simulink library "LIB_CycleControl"  (R2018b)
settings: Solver=VariableStepAuto  StartTime=0.0  StopTime=10.0  RelTol=1e-3
undefined symbols (not defined in the file or in its folder): eActuators, eRespiratorStates, NActuatorActive, nBlowerCmdInit, nBlowerCmdMax, nBlowerCmdMin, nBlowerDecHigh, nBlowerDecMedium, nBlowerIncHigh, nBlowerIncLow, nBlowerIncMedium, NBlowerSpeedIncCorrectionGain, NBlowerValveDerivativeGain, NBlowerValveIntegralGain, NBlowerValveIntegralHighGain, NBlowerValvePropGain, NCyclePerMinMax, NCyclePerMinMin, NMaxPressureSample, NPatientValveDerivativeGain, NPatientValveIntegralGain, NPatientValveIntegralHighGain, NPatientValvePropGain, pBlowerValveOutletOffset, pDiffMaxThdForPlateauPlausibility, pDiffThdForBlowerValveControlActivation, pDiffThdForPatientValveControlActivation, pErrorPlausibilityThd, pErrorThdForHighBlowerDec, pStaticErrorThdForHighBlowerInc, rPIDIntegralMaxTermForBlowerValve, rPIDIntegralMaxTermForPatientValve, rPIDIntegralMinTermForBlowerValve, rPIDIntegralMinTermForPatientValve, tBlowerValveOpen, tDelayBeforeRespiratorCycleStart, tDelayForRespiratorStop, tPatientValveOpen, tPhase1Ofs, tStopInhalationPhase1Min
libraries: simulink x62, simulink_need_slupdate x4, simulink_extras x3
(part 2 of 4)

== system LIB_CycleControl/Cycle Control/Cycle Control Wrapper/Cycle pController/Pressure processing/PPep Computation ==
  BInitCyclePressure [-] : Inport
  NRespiratorCycleStatus [-] : Inport  Port=2
  pBlowerValveOutletLastValuesMean [mmH2O] : Inport  Port=3
  Compare To Constant4 : simulink/Logic and Bit Operations/Compare To Constant  relop===  const=eRespiratorStates.NRespiratorInExhalation  OutDataTypeStr=boolean
  Data Store Write1 : DataStoreWrite  DataStoreName=pBlowerValveOutletExhalationCurrent
  Logical Operator7 : Logic  Operator=OR  AllPortsSameDT=off  OutDataTypeStr=boolean
  PPep Computation : Subsystem
  pBlowerValveOutletExhalationCurrent [mmH2O] : Outport
  wires:
  pBlowerValveOutletLastValuesMean [mmH2O]/1 -> PPep Computation/2(pBlowerValveOutletLastValuesMean [mmH2O])
  BInitCyclePressure [-]/1 -> Logical Operator7/2, PPep Computation/1(BInitCyclePressure [-])
  Compare To Constant4/1 -> Logical Operator7/1
  Logical Operator7/1 -> PPep Computation/Enable
  PPep Computation/1(pBlowerValveOutletExhalationCurrent [mmH2O]) -> pBlowerValveOutletExhalationCurrent [mmH2O]/1, Data Store Write1/1  "pBlowerValveOutletExhalationCurrent"
  NRespiratorCycleStatus [-]/1 -> Compare To Constant4/1

== system LIB_CycleControl/Cycle Control/Cycle Control Wrapper/Cycle pController/Pressure processing/PPlateau Computation ==
  BInitCyclePressure [-] : Inport
  NRespiratorCycleStatus [-] : Inport  Port=2
  pBlowerValveOutletLastValuesMax [mmH2O] : Inport  Port=3
  pBlowerValveOutletLastValuesMin [mmH2O] : Inport  Port=4
  pBlowerValveOutletLastValuesMean [mmH2O] : Inport  Port=5
  Compare To Constant6 : simulink/Logic and Bit Operations/Compare To Constant  relop===  const=eRespiratorStates.NRespiratorInInhalationPhase2  OutDataTypeStr=boolean
  Data Store Write1 : DataStoreWrite  DataStoreName=BpBlowerValveOutletPlateauStabilized
  Data Store Write3 : DataStoreWrite  DataStoreName=pBlowerValveOutletPlateauCurrent
  Logical Operator7 : Logic  Operator=OR  AllPortsSameDT=off  OutDataTypeStr=boolean
  Plateau Compute : Subsystem
  pBlowerValveOutletPlateauCurrent [mmH2O] : Outport
  BpBlowerValveOutletPlateauStabilized [-] : Outport  Port=2
  wires:
  Plateau Compute/2(BpBlowerValveOutletPlateauStabilized [-]) -> BpBlowerValveOutletPlateauStabilized [-]/1, Data Store Write1/1  "BpBlowerValveOutletPlateauStabilized"
  pBlowerValveOutletLastValuesMean [mmH2O]/1 -> Plateau Compute/4(pBlowerValveOutletLastValuesMean [mmH2O])
  pBlowerValveOutletLastValuesMin [mmH2O]/1 -> Plateau Compute/3(pBlowerValveOutletLastValuesMin [mmH2O])
  pBlowerValveOutletLastValuesMax [mmH2O]/1 -> Plateau Compute/2(pBlowerValveOutletLastValuesMax [mmH2O])
  Logical Operator7/1 -> Plateau Compute/Enable
  Compare To Constant6/1 -> Logical Operator7/2
  [BInitCyclePressure] -> Plateau Compute/1(BInitCyclePressure [-])
  NRespiratorCycleStatus [-]/1 -> Compare To Constant6/1
  [BInitCyclePressure] -> Logical Operator7/1
  BInitCyclePressure [-]/1 -> [BInitCyclePressure]
  Plateau Compute/1(pBlowerValveOutletPlateauCurrent [mmH2O]) -> pBlowerValveOutletPlateauCurrent [mmH2O]/1, Data Store Write3/1  "pBlowerValveOutletPlateauCurrent"

== system LIB_CycleControl/Cycle Control/Cycle Control Wrapper/Cycle pController/Pressure processing/PPlateau Error Max Computation ==
  BInitCyclePressure [-] : Inport
  NRespiratorCycleStatus [-] : Inport  Port=2
  pBlowerValveOutletPeakCurrent [mmH2O] : Inport  Port=3
  pBlowerValveOutlet [mmH2O] : Inport  Port=4
  pBlowerValveOutletPlateauTargetApplied [mmH2O] : Inport  Port=5
  Compare To Constant6 : simulink/Logic and Bit Operations/Compare To Constant  relop===  const=eRespiratorStates.NRespiratorInInhalationPhase2  OutDataTypeStr=boolean
  Data Store Write3 : DataStoreWrite  DataStoreName=pBlowerValveOutletErrorMaxCurrent
  Error Compute : Subsystem
  Logical Operator1 : Logic  AllPortsSameDT=off  OutDataTypeStr=boolean
  Logical Operator7 : Logic  Operator=OR  AllPortsSameDT=off  OutDataTypeStr=boolean
  Relational Operator : RelationalOperator  Operator=>  OutDataTypeStr=boolean  RndMeth=Simplest
  Unit Delay : UnitDelay  SampleTime=-1
      settings: AttributesFormatString=%<InitialCondition>
  pBlowerValveOutletErrorMaxCurrent [mmH2O] : Outport
  wires:
  [pBlowerValveOutlet] -> Error Compute/3(pBlowerValveOutlet [mmH2O])
  Unit Delay/1 -> Error Compute/4(pBlowerValveOutletErrorMaxCurrentPrev [mmH2O])
  [pBlowerValveOutletPlateauTargetApplied] -> Error Compute/2(pBlowerValveOutletPlateauTargetApplied [mmH2O])
  Relational Operator/1 -> Logical Operator1/2
  [pBlowerValveOutletPeakCurrent] -> Relational Operator/1
  [pBlowerValveOutletPlateauTargetApplied] -> Relational Operator/2
  pBlowerValveOutletPeakCurrent [mmH2O]/1 -> [pBlowerValveOutletPeakCurrent]
  pBlowerValveOutletPlateauTargetApplied [mmH2O]/1 -> [pBlowerValveOutletPlateauTargetApplied]
  Logical Operator1/1 -> Logical Operator7/2
  Compare To Constant6/1 -> Logical Operator1/1
  pBlowerValveOutlet [mmH2O]/1 -> [pBlowerValveOutlet]
  Logical Operator7/1 -> Error Compute/Enable
  [BInitCyclePressure] -> Error Compute/1(BInitCyclePressure [-])
  NRespiratorCycleStatus [-]/1 -> Compare To Constant6/1
  [BInitCyclePressure] -> Logical Operator7/1
  BInitCyclePressure [-]/1 -> [BInitCyclePressure]
  Error Compute/1(pBlowerValveOutletErrorMaxCurrent [mmH2O]) -> pBlowerValveOutletErrorMaxCurrent [mmH2O]/1, Data Store Write3/1, Unit Delay/1  "pBlowerValveOutletErrorMaxCurrent"

== system LIB_CycleControl/Cycle Control/Cycle Control Wrapper/Cycle pController/Pressure processing/Pressure Release  ==
  NRespiratorCycleStatus [-] : Inport
  BInitCyclePressure [-] : Inport  Port=2
  pBlowerValveOutletPeakCurrentPrev [mmH2O] : Inport  Port=3
  pBlowerValveOutletErrorMaxCurrentPrev [mmH2O] : Inport  Port=4
  pBlowerValveOutletPlateauCurrentPrev [mmH2O] : Inport  Port=5
  BpBlowerValveOutletPlateauStabilizedPrev [-] : Inport  Port=6
  pBlowerValveOutletExhalationCurrentPrev [mmH2O] : Inport  Port=7
  Release : Subsystem
  pBlowerValveOutletPeakLastCycle [mmH2O] : Outport
  pBlowerValveOutletPlateauLastCycle [mmH2O] : Outport  Port=2  InitialOutput=0
  pBlowerValveOutletEndLastCycle [mmH2O] : Outport  Port=3
  pBlowerValveOutletErrorMaxLastCycle [mmH2O] : Outport  Port=4  InitialOutput=0
  wires:
  Release/3(pBlowerValveOutletEndLastCycle [mmH2O]) -> pBlowerValveOutletEndLastCycle [mmH2O]/1
  Release/1(pBlowerValveOutletPeakLastCycle [mmH2O]) -> pBlowerValveOutletPeakLastCycle [mmH2O]/1
  BpBlowerValveOutletPlateauStabilizedPrev [-]/1 -> Release/6(BpBlowerValveOutletPlateauStabilizedPrev [-])
  pBlowerValveOutletErrorMaxCurrentPrev [mmH2O]/1 -> Release/5(pBlowerValveOutletErrorMaxCurrentPrev [mmH2O])
  Release/4(pBlowerValveOutletErrorMaxLastCycle [mmH2O]) -> pBlowerValveOutletErrorMaxLastCycle [mmH2O]/1
  BInitCyclePressure [-]/1 -> Release/Enable
  Release/2(pBlowerValveOutletPlateauLastCycle [mmH2O]) -> pBlowerValveOutletPlateauLastCycle [mmH2O]/1
  pBlowerValveOutletExhalationCurrentPrev [mmH2O]/1 -> Release/4(pBlowerValveOutletExhalationCurrentPrev [mmH2O])
  pBlowerValveOutletPlateauCurrentPrev [mmH2O]/1 -> Release/3(pBlowerValveOutletPlateauCurrentPrev [mmH2O])
  pBlowerValveOutletPeakCurrentPrev [mmH2O]/1 -> Release/2(pBlowerValveOutletPeakCurrentPrev [mmH2O])
  NRespiratorCycleStatus [-]/1 -> Release/1(NRespiratorCycleStatus [-])

== system LIB_CycleControl/Cycle Control/Cycle Control Wrapper/Cycle pController/Pressure processing/Pressure recording Update ==
  note: [0...NSample-1]
  pBlowerValveOutlet [mmH2O] : Inport
  BInitCyclePressure [-] : Inport  Port=2
  Assignment : Assignment  IndexMode=Zero-based  DiagnosticForDimensions=Warning  IndexOptions=Index vector (port)  Indices=1  OutputSizes=1
      settings: AttributesFormatString=%<IndexMode>
  Constant : Constant  Value=zeros(1,NMaxPressureSample)  OutDataTypeStr=single
  Constant1 : Constant  Value=NMaxPressureSample
  Counter : Subsystem
  Data Store Write1 : DataStoreWrite  DataStoreName=pBlowerValveOutletLastValuesMin
  Data Store Write2 : DataStoreWrite  DataStoreName=pBlowerValveOutletLastValuesMax
  Data Store Write3 : DataStoreWrite  DataStoreName=pBlowerValveOutletLastValuesMean
  MinMax : MinMax  Function=max
  MinMax1 : MinMax
  Product : Product  Inputs=*/
  Sum of Elements : Sum  Inputs=+
  Switch4 : Switch  Criteria=u2 ~= 0
      settings: AttributesFormatString=%<Criteria>
  Unit Delay : UnitDelay  InitialCondition=zeros(1,NMaxPressureSample)  SampleTime=-1
      settings: AttributesFormatString=%<InitialCondition>
  pBlowerValveOutletLastValuesMax [mmH2O] : Outport
  pBlowerValveOutletLastValuesMin [mmH2O] : Outport  Port=2
  pBlowerValveOutletLastValuesMean [mmH2O] : Outport  Port=3
  wires:
  Product/1 -> pBlowerValveOutletLastValuesMean [mmH2O]/1, Data Store Write3/1  "pBlowerValveOutletLastValuesMean"
  MinMax1/1 -> pBlowerValveOutletLastValuesMin [mmH2O]/1, Data Store Write1/1  "pBlowerValveOutletLastValuesMin"
  MinMax/1 -> pBlowerValveOutletLastValuesMax [mmH2O]/1, Data Store Write2/1  "pBlowerValveOutletLastValuesMax"
  Constant1/1 -> Product/2
  Sum of Elements/1 -> Product/1
  pBlowerValveOutlet [mmH2O]/1 -> Assignment/2
  Counter/1(NPressureSampleIndex [-]) -> Assignment/3
  Constant/1 -> Switch4/1
  BInitCyclePressure [-]/1 -> Switch4/2
  Switch4/1 -> MinMax1/1, Sum of Elements/1, Unit Delay/1, MinMax/1
  Assignment/1 -> Switch4/3
  Unit Delay/1 -> Assignment/1

== system LIB_CycleControl/Cycle Control/Cycle Control Wrapper/Cycle pController/ValvePosition_Target/Exhalation ==
  BExternalInit [-] : Inport
  tPeriodTask [s] : Inport  Port=2
  pBlowerValveOutletTarget [mmH2O] : Inport  Port=3
  pBlowerValveOutlet [mmH2O] : Inport  Port=4
  rPatientValveCmdPrev [%] : Inport  Port=5
  Action Port : ActionPort
  Constant2 : Constant  Value=0  OutDataTypeStr=Inherit: Inherit via back propagation
  Patient Valve Control : Subsystem
  Sum : Sum  Inputs=|+-  SaturateOnIntegerOverflow=on
  rBlowerValveCmd [%] : Outport
  rPatientValveCmd [%] : Outport  Port=2
  wires:
  Sum/1 -> Patient Valve Control/4(Error [mmH2O])
  rPatientValveCmdPrev [%]/1 -> Patient Valve Control/5(rPatientValveCmdPrev [%])
  Patient Valve Control/1(rPatientValveCmd [%]) -> rPatientValveCmd [%]/1
  BExternalInit [-]/1 -> Patient Valve Control/2(BExternalInit [-])
  pBlowerValveOutletTarget [mmH2O]/1 -> Sum/1, Patient Valve Control/3(pBlowerValveOutletTarget [mmH2O])
  pBlowerValveOutlet [mmH2O]/1 -> Sum/2
  tPeriodTask [s]/1 -> Patient Valve Control/1(tPeriodTask [s])
  Constant2/1 -> rBlowerValveCmd [%]/1

== system LIB_CycleControl/Cycle Control/Cycle Control Wrapper/Cycle pController/ValvePosition_Target/Inhalation ==
  BExternalInit [-] : Inport
  tPeriodTask [s] : Inport  Port=2
  pBlowerValveOutletTarget [mmH2O] : Inport  Port=3
  pBlowerValveOutlet [mmH2O] : Inport  Port=4
  rBlowerValveCmdPrev [%] : Inport  Port=5
  Action Port : ActionPort
  Blower Valve Control : Subsystem
  Constant9 : Constant  Value=0  OutDataTypeStr=single
  Sum : Sum  Inputs=|+-  SaturateOnIntegerOverflow=on
  rBlowerValveCmd [%] : Outport
  rPatientValveCmd [%] : Outport  Port=2
  wires:
  rBlowerValveCmdPrev [%]/1 -> Blower Valve Control/4(rBlowerValveCmdPrev [%])
  Sum/1 -> Blower Valve Control/3(Error)
  Blower Valve Control/1(rBlowerValveCmd [%]) -> rBlowerValveCmd [%]/1
  pBlowerValveOutlet [mmH2O]/1 -> Sum/2
  tPeriodTask [s]/1 -> Blower Valve Control/1(tPeriodTask [s])
  pBlowerValveOutletTarget [mmH2O]/1 -> Sum/1
  BExternalInit [-]/1 -> Blower Valve Control/2(BExternalInit [-])
  Constant9/1 -> rPatientValveCmd [%]/1

== system LIB_CycleControl/Cycle Control/Cycle Control Wrapper/Cycle pController/ValvePosition_Target/START ==
  Action Port : ActionPort
  Constant2 : Constant  Value=0  OutDataTypeStr=Inherit: Inherit via back propagation
  Constant9 : Constant  Value=100  OutDataTypeStr=Inherit: Inherit via back propagation
  rBlowerValveCmd [%] : Outport
  rPatientValveCmd [%] : Outport  Port=2
  wires:
  Constant2/1 -> rBlowerValveCmd [%]/1
  Constant9/1 -> rPatientValveCmd [%]/1

== system LIB_CycleControl/Cycle Control/Cycle Control Wrapper/Cycle pController/ValvePosition_Target/STOP ==
  tCycle [s] : Inport
  Action Port : ActionPort
  Constant1 : Constant  Value=100  OutDataTypeStr=Inherit: Inherit via back propagation
  Constant2 : Constant  Value=0  OutDataTypeStr=Inherit: Inherit via back propagation
  Constant3 : Constant  Value=tDelayForRespiratorStop  OutDataTypeStr=single
  Constant9 : Constant  Value=100  OutDataTypeStr=single
  Gain : Gain  Gain=0.5
  Relational Operator : RelationalOperator  Operator=>  OutDataTypeStr=boolean  RndMeth=Simplest
  Switch3 : Switch  Criteria=u2 ~= 0
      settings: AttributesFormatString=%<Criteria>
  rBlowerValveCmd [%] : Outport
  rPatientValveCmd [%] : Outport  Port=2
  wires:
  Constant3/1 -> Gain/1
  Constant2/1 -> Switch3/3
  Constant1/1 -> rPatientValveCmd [%]/1
  Gain/1 -> Relational Operator/2
  Switch3/1 -> rBlowerValveCmd [%]/1
  Constant9/1 -> Switch3/1
  Relational Operator/1 -> Switch3/2
  tCycle [s]/1 -> Relational Operator/1

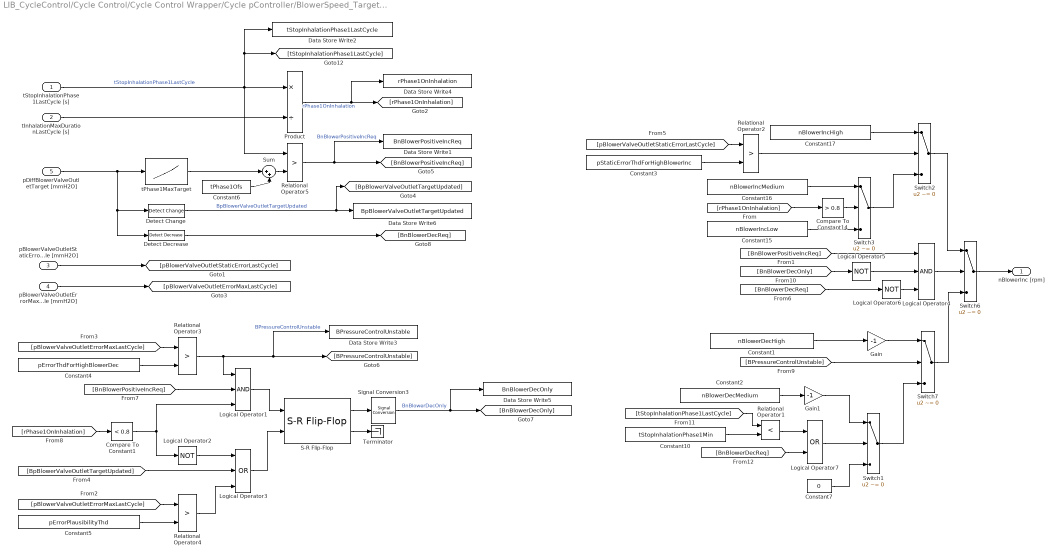
== system LIB_CycleControl/Cycle Control/Cycle Control Wrapper/Cycle pController/BlowerSpeed_Target/CycleStartComputation/Blower Inc from Last Cycle ==
  tStopInhalationPhase1LastCycle [s] : Inport
  tInhalationMaxDurationLastCycle [s] : Inport  Port=2
  "pBlowerValveOutletStaticErrorLastCycle [mmH2O] " : Inport  Port=3
  pBlowerValveOutletErrorMaxLastCycle [mmH2O] : Inport  Port=4
  pDiffBlowerValveOutletTarget [mmH2O] : Inport  Port=5
  Compare To Constant1 : simulink/Logic and Bit Operations/Compare To Constant  relop=<  const=0.8  OutDataTypeStr=boolean
  Compare To Constant14 : simulink/Logic and Bit Operations/Compare To Constant  relop=>  const=0.8  OutDataTypeStr=boolean
  Constant1 : Constant  Value=nBlowerDecHigh  OutDataTypeStr=single
  Constant10 : Constant  Value=tStopInhalationPhase1Min  OutDataTypeStr=single
  Constant15 : Constant  Value=nBlowerIncLow  OutDataTypeStr=single
  Constant16 : Constant  Value=nBlowerIncMedium  OutDataTypeStr=single
  Constant17 : Constant  Value=nBlowerIncHigh  OutDataTypeStr=single
  Constant2 : Constant  Value=nBlowerDecMedium  OutDataTypeStr=single
  Constant3 : Constant  Value=pStaticErrorThdForHighBlowerInc  OutDataTypeStr=single
  Constant4 : Constant  Value=pErrorThdForHighBlowerDec  OutDataTypeStr=single
  Constant5 : Constant  Value=pErrorPlausibilityThd  OutDataTypeStr=single
  Constant6 : Constant  Value=tPhase1Ofs  OutDataTypeStr=single
  Constant7 : Constant  Value=0  OutDataTypeStr=single
  Data Store Write1 : DataStoreWrite  DataStoreName=BnBlowerPositiveIncReq
  Data Store Write2 : DataStoreWrite  DataStoreName=tStopInhalationPhase1LastCycle
  Data Store Write3 : DataStoreWrite  DataStoreName=BPressureControlUnstable
  Data Store Write4 : DataStoreWrite  DataStoreName=rPhase1OnInhalation
  Data Store Write5 : DataStoreWrite  DataStoreName=BnBlowerDecOnly
  Data Store Write6 : DataStoreWrite  DataStoreName=BpBlowerValveOutletTargetUpdated
  Detect Change : simulink/Logic and Bit Operations/Detect Change  vinit=0  OutDataTypeStr=boolean
  Detect Decrease : simulink/Logic and Bit Operations/Detect Decrease  vinit=0.0  OutDataTypeStr=boolean
  Gain : Gain  Gain=-1
  Gain1 : Gain  Gain=-1
  Logical Operator1 : Logic  Inputs=3  AllPortsSameDT=off  OutDataTypeStr=boolean
  Logical Operator2 : Logic  Operator=NOT  Inputs=3  AllPortsSameDT=off  OutDataTypeStr=boolean
  Logical Operator3 : Logic  Operator=OR  Inputs=3  AllPortsSameDT=off  OutDataTypeStr=boolean
  Logical Operator4 : Logic  Inputs=3  AllPortsSameDT=off  OutDataTypeStr=boolean
  Logical Operator5 : Logic  Operator=NOT  Inputs=3  AllPortsSameDT=off  OutDataTypeStr=boolean
  Logical Operator6 : Logic  Operator=NOT  Inputs=3  AllPortsSameDT=off  OutDataTypeStr=boolean
  Logical Operator7 : Logic  Operator=OR  AllPortsSameDT=off  OutDataTypeStr=boolean
  Product : Product  Inputs=*/
  Relational Operator1 : RelationalOperator  Operator=<  OutDataTypeStr=boolean  RndMeth=Simplest
  Relational Operator{2..5} (4 alike) : RelationalOperator  Operator=>  OutDataTypeStr=boolean  RndMeth=Simplest
  S-R Flip-Flop : simulink_extras/Flip Flops/S-R Flip-Flop  initial_condition=0
  Signal Conversion3 : SignalConversion  OverrideOpt=off
  Sum : Sum  Inputs=|++
  Switch{1..3,6..7} (5 alike) : Switch  Criteria=u2 ~= 0
      settings: AttributesFormatString=%<Criteria>
  Terminator : Terminator
  tPhase1MaxTarget : Lookup_n-D  NumberOfTableDimensions=1  BreakpointsForDimension1=[50 100 150 200 250 350]  IndexSearchMethod=Linear search  BeginIndexSearchUsingPreviousIndexResult=on  Table=[0.225 0.275 0.35 0.425 0.55 0.8]  ExtrapMethod=Clip  UseLastTableValue=on  InternalRulePriority=Speed  RndMeth=Simplest  InputSameDT=on
  nBlowerInc [rpm] : Outport
  wires:
  Constant6/1 -> Sum/2
  Sum/1 -> Relational Operator5/2
  tPhase1MaxTarget/1 -> Sum/1
  [BnBlowerDecReq] -> Logical Operator7/2
  Relational Operator1/1 -> Logical Operator7/1
  Logical Operator7/1 -> Switch1/2
  [BPressureControlUnstable] -> Switch7/2
  [BnBlowerDecReq] -> Logical Operator6/1
  Logical Operator6/1 -> Logical Operator4/3
  Detect Decrease/1 -> [BnBlowerDecReq]
  [BpBlowerValveOutletTargetUpdated] -> Logical Operator3/2
  Detect Change/1 -> Data Store Write6/1, [BpBlowerValveOutletTargetUpdated]  "BpBlowerValveOutletTargetUpdated"
  pDiffBlowerValveOutletTarget [mmH2O]/1 -> tPhase1MaxTarget/1, Detect Decrease/1, Detect Change/1
  Signal Conversion3/1 -> [BnBlowerDecOnly], Data Store Write5/1  "BnBlowerDecOnly"
  Relational Operator5/1 -> [BnBlowerPositiveIncReq], Data Store Write1/1  "BnBlowerPositiveIncReq"
  Logical Operator4/1 -> Switch6/2
  [BnBlowerDecOnly] -> Logical Operator5/1
  Logical Operator5/1 -> Logical Operator4/2
  [BnBlowerPositiveIncReq] -> Logical Operator4/1
  Constant5/1 -> Relational Operator4/2
  S-R Flip-Flop/2 -> Terminator/1
  Relational Operator4/1 -> Logical Operator3/3
  [pBlowerValveOutletErrorMaxLastCycle] -> Relational Operator4/1
  Logical Operator3/1 -> S-R Flip-Flop/2
  Logical Operator2/1 -> Logical Operator3/1
  Compare To Constant1/1 -> Logical Operator2/1, Logical Operator1/3
  [BnBlowerPositiveIncReq] -> Logical Operator1/2
  Logical Operator1/1 -> S-R Flip-Flop/1
  [rPhase1OnInhalation] -> Compare To Constant1/1
  Relational Operator3/1 -> [BPressureControlUnstable], Data Store Write3/1, Logical Operator1/1  "BPressureControlUnstable"
  S-R Flip-Flop/1 -> Signal Conversion3/1
  Constant4/1 -> Relational Operator3/2
  [pBlowerValveOutletErrorMaxLastCycle] -> Relational Operator3/1
  Constant3/1 -> Relational Operator2/2
  tInhalationMaxDurationLastCycle [s]/1 -> Product/2
  tStopInhalationPhase1LastCycle [s]/1 -> Relational Operator5/1, Product/1, [tStopInhalationPhase1LastCycle], Data Store Write2/1  "tStopInhalationPhase1LastCycle"
  Product/1 -> [rPhase1OnInhalation], Data Store Write4/1  "rPhase1OnInhalation"
  pBlowerValveOutletErrorMaxLastCycle [mmH2O]/1 -> [pBlowerValveOutletErrorMaxLastCycle]
  Constant10/1 -> Relational Operator1/2
  Constant1/1 -> Gain/1
  Constant2/1 -> Gain1/1
  Constant15/1 -> Switch3/3
  Constant16/1 -> Switch3/1
  Constant17/1 -> Switch2/1
  Relational Operator2/1 -> Switch2/2
  Switch3/1 -> Switch2/3
  Switch2/1 -> Switch6/1
  [pBlowerValveOutletStaticErrorLastCycle] -> Relational Operator2/1
  Gain1/1 -> Switch1/1
  [tStopInhalationPhase1LastCycle] -> Relational Operator1/1
  Constant7/1 -> Switch1/3
  Gain/1 -> Switch7/1
  Switch1/1 -> Switch7/3
  Switch7/1 -> Switch6/3
  [rPhase1OnInhalation] -> Compare To Constant14/1
  Switch6/1 -> nBlowerInc [rpm]/1
  Compare To Constant14/1 -> Switch3/2
  "pBlowerValveOutletStaticErrorLastCycle [mmH2O] "/1 -> [pBlowerValveOutletStaticErrorLastCycle]

== system LIB_CycleControl/Cycle Control/Cycle Control Wrapper/Cycle pController/BlowerSpeed_Target/CycleStartComputation/Saturation Dynamic with flags ==
  up : Inport
  u : Inport  Port=2
  lo : Inport  Port=3
  Data Type Duplicate : DataTypeDuplicate
  Data Type Propagation : simulink/Signal Attributes/Data Type Propagation  PropDataType=fixdt(1, 16)  IfRefDouble=double  IfRefSingle=single  IsSigned=IsSigned1  NumBitsBase=NumBits1  NumBitsMult=1  NumBitsAdd=0  NumBitsAllowFinal=1:128  PropScaling=2^-10  ValuesUsedBestPrec=[5 -7]  SlopeBase=Slope1  SlopeMult=1  SlopeAdd=0  BiasBase=Bias1  BiasMult=1  BiasAdd=0
      settings: SourceProductName=Simulink  SourceProductBaseCode=SL
  LowerRelop1 : RelationalOperator  DisableCoverage=on  Operator=>  OutDataTypeStr=boolean  RndMeth=Nearest
  Switch : Switch  Criteria=u2 ~= 0  OutDataTypeStr=Inherit: Inherit via back propagation  ZeroCross=off
  Switch2 : Switch  Criteria=u2 ~= 0  OutMin=OutMin  OutMax=OutMax  OutDataTypeStr=Inherit: Inherit via back propagation  ZeroCross=off
  UpperRelop : RelationalOperator  DisableCoverage=on  Operator=<  OutDataTypeStr=boolean  RndMeth=Nearest
  BsatUp [-] : Outport  OutMin=OutMin  OutMax=OutMax
  y : Outport  Port=2  OutMin=OutMin  OutMax=OutMax
  BsatDown [-] : Outport  Port=3  OutMin=OutMin  OutMax=OutMax
  wires:
  up/1 -> Switch2/1, LowerRelop1/2
  u/1 -> Data Type Propagation/2, Data Type Propagation/1, LowerRelop1/1, Switch/3, UpperRelop/1
  lo/1 -> Switch/1, UpperRelop/2
  Switch/1 -> Data Type Duplicate/2, Switch2/3, Data Type Propagation/3
  Switch2/1 -> Data Type Duplicate/1, y/1
  LowerRelop1/1 -> Switch2/2, BsatUp [-]/1
  UpperRelop/1 -> BsatDown [-]/1, Switch/2

== system LIB_CycleControl/Cycle Control/Cycle Control Wrapper/Cycle pController/Cycle Manager/Timing Setup/Timing Setup ==
  NCyclePerMin [-/min] : Inport
  rInhalationPerCycle : Inport  Port=2
  Constant2 : Constant  Value=0  OutDataTypeStr=single
  Constant6 : Constant  Value=60  OutDataTypeStr=single
  Product : Product  Inputs=*/
  Product1 : Product  Inputs=**
  Saturation1 : Saturate  UpperLimit=NCyclePerMinMax  LowerLimit=NCyclePerMinMin
      settings: AttributesFormatString=|
      | %<UpperLimit>
      | %<LowerLimit>
  Switch4 : Switch  Criteria=u2 ~= 0
      settings: AttributesFormatString=%<Criteria>
  Unit Delay1 : UnitDelay  InitialCondition=1  SampleTime=-1
      settings: AttributesFormatString=%<InitialCondition>
  Unit Delay2 : UnitDelay  InitialCondition=1  SampleTime=-1
      settings: AttributesFormatString=%<InitialCondition>
  tCycleMaxDuration [s] : Outport
  tInhalationMaxDuration [s] : Outport  Port=2
  tInhalationMaxDurationLastCycle [s] : Outport  Port=3
  wires:
  Switch4/1 -> tInhalationMaxDurationLastCycle [s]/1
  Unit Delay2/1 -> Switch4/3
  Unit Delay1/1 -> Switch4/2
  Product1/1 -> Switch4/1, Unit Delay2/1, tInhalationMaxDuration [s]/1
  Constant2/1 -> Unit Delay1/1
  Product/1 -> Product1/1, tCycleMaxDuration [s]/1
  NCyclePerMin [-/min]/1 -> Saturation1/1
  rInhalationPerCycle/1 -> Product1/2
  Constant6/1 -> Product/1
  Saturation1/1 -> Product/2

== system LIB_CycleControl/Cycle Control/Cycle Control Wrapper/Cycle pController/Pressure Target/CycleStartComputation/Update_PlateauError ==
  NRespiratorCycleStatus [-] : Inport
  pBlowerValveOutletPlateauTargetAppliedLastCycle [mmH2O] : Inport  Port=2  OutDataTypeStr=single
  pBlowerValveOutletPlateauLastCycle [mmH2O] : Inport  Port=3
  Enable : EnablePort
  Compare To Constant1 : simulink/Logic and Bit Operations/Compare To Constant  relop===  const=eRespiratorStates.NRespiratorStart  OutDataTypeStr=boolean
  Compare To Constant3 : simulink/Logic and Bit Operations/Compare To Constant  relop===  const=eRespiratorStates.NRespiratorStop  OutDataTypeStr=boolean
  Constant5 : Constant  Value=0  OutDataTypeStr=single
  Data Store Write4 : DataStoreWrite  DataStoreName=pBlowerValveOutletStaticErrorLastCycle
  Logical Operator : Logic  Operator=OR  AllPortsSameDT=off  OutDataTypeStr=boolean
  Sum4 : Sum  Inputs=|+-
  Switch2 : Switch  Criteria=u2 ~= 0
      settings: AttributesFormatString=%<Criteria>
  pBlowerValveOutletStaticErrorLastCycle [mmH2O] : Outport
  wires:
  pBlowerValveOutletPlateauLastCycle [mmH2O]/1 -> Sum4/2
  pBlowerValveOutletPlateauTargetAppliedLastCycle [mmH2O]/1 -> Sum4/1
  Switch2/1 -> pBlowerValveOutletStaticErrorLastCycle [mmH2O]/1, Data Store Write4/1  "pBlowerValveOutletStaticErrorLastCycle"
  Compare To Constant1/1 -> Logical Operator/1
  Constant5/1 -> Switch2/1
  Logical Operator/1 -> Switch2/2
  NRespiratorCycleStatus [-]/1 -> Compare To Constant3/1, Compare To Constant1/1
  Compare To Constant3/1 -> Logical Operator/2
  Sum4/1 -> Switch2/3

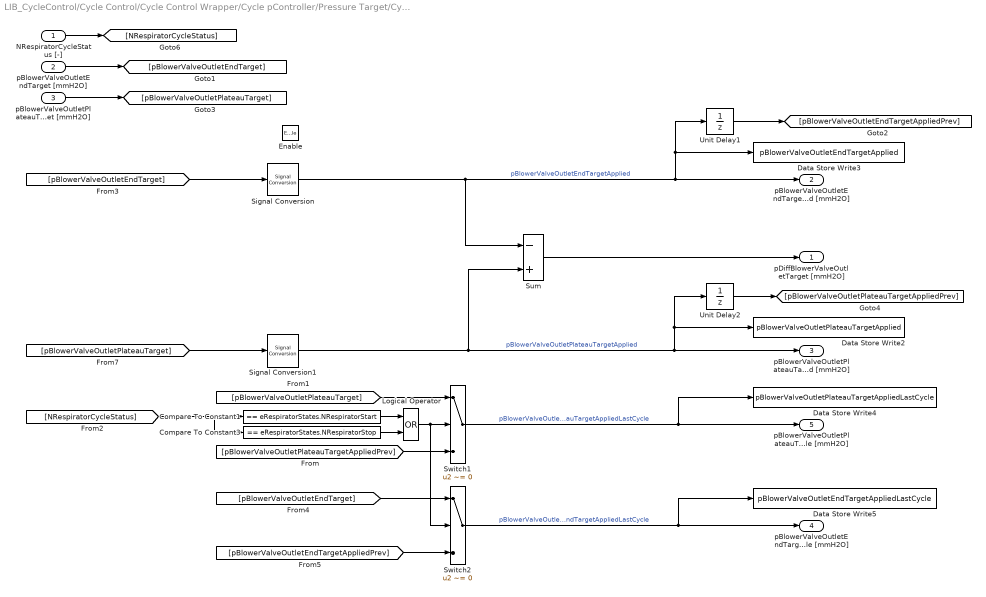
== system LIB_CycleControl/Cycle Control/Cycle Control Wrapper/Cycle pController/Pressure Target/CycleStartComputation/Update_Pressure ==
  NRespiratorCycleStatus [-] : Inport
  pBlowerValveOutletEndTarget [mmH2O] : Inport  Port=2
  pBlowerValveOutletPlateauTarget [mmH2O] : Inport  Port=3
  Enable : EnablePort
  Compare To Constant1 : simulink/Logic and Bit Operations/Compare To Constant  relop===  const=eRespiratorStates.NRespiratorStart  OutDataTypeStr=boolean
  Compare To Constant3 : simulink/Logic and Bit Operations/Compare To Constant  relop===  const=eRespiratorStates.NRespiratorStop  OutDataTypeStr=boolean
  Data Store Write2 : DataStoreWrite  DataStoreName=pBlowerValveOutletPlateauTargetApplied
  Data Store Write3 : DataStoreWrite  DataStoreName=pBlowerValveOutletEndTargetApplied
  Data Store Write4 : DataStoreWrite  DataStoreName=pBlowerValveOutletPlateauTargetAppliedLastCycle
  Data Store Write5 : DataStoreWrite  DataStoreName=pBlowerValveOutletEndTargetAppliedLastCycle
  Logical Operator : Logic  Operator=OR  AllPortsSameDT=off  OutDataTypeStr=boolean
  Signal Conversion : SignalConversion  OverrideOpt=off
  Signal Conversion1 : SignalConversion  OverrideOpt=off
  Sum : Sum  Inputs=-+
  Switch1 : Switch  Criteria=u2 ~= 0
      settings: AttributesFormatString=%<Criteria>
  Switch2 : Switch  Criteria=u2 ~= 0
      settings: AttributesFormatString=%<Criteria>
  Unit Delay1 : UnitDelay  SampleTime=-1
      settings: AttributesFormatString=%<InitialCondition>
  Unit Delay2 : UnitDelay  SampleTime=-1
      settings: AttributesFormatString=%<InitialCondition>
  pDiffBlowerValveOutletTarget [mmH2O] : Outport
  pBlowerValveOutletEndTargetApplied [mmH2O] : Outport  Port=2
  pBlowerValveOutletPlateauTargetApplied [mmH2O] : Outport  Port=3
  pBlowerValveOutletEndTargetAppliedLastCycle [mmH2O] : Outport  Port=4
  pBlowerValveOutletPlateauTargetAppliedLastCycle [mmH2O] : Outport  Port=5
  wires:
  Unit Delay2/1 -> [pBlowerValveOutletPlateauTargetAppliedPrev]
  [pBlowerValveOutletEndTargetAppliedPrev] -> Switch2/3
  Unit Delay1/1 -> [pBlowerValveOutletEndTargetAppliedPrev]
  Switch2/1 -> pBlowerValveOutletEndTargetAppliedLastCycle [mmH2O]/1, Data Store Write5/1  "pBlowerValveOutletEndTargetAppliedLastCycle"
  [pBlowerValveOutletEndTarget] -> Switch2/1
  [pBlowerValveOutletEndTarget] -> Signal Conversion/1
  pBlowerValveOutletEndTarget [mmH2O]/1 -> [pBlowerValveOutletEndTarget]
  [NRespiratorCycleStatus] -> Compare To Constant1/1, Compare To Constant3/1
  NRespiratorCycleStatus [-]/1 -> [NRespiratorCycleStatus]
  Sum/1 -> pDiffBlowerValveOutletTarget [mmH2O]/1
  [pBlowerValveOutletPlateauTargetAppliedPrev] -> Switch1/3
  Signal Conversion1/1 -> pBlowerValveOutletPlateauTargetApplied [mmH2O]/1, Data Store Write2/1, Unit Delay2/1, Sum/2  "pBlowerValveOutletPlateauTargetApplied"
  Signal Conversion/1 -> Sum/1, pBlowerValveOutletEndTargetApplied [mmH2O]/1, Data Store Write3/1, Unit Delay1/1  "pBlowerValveOutletEndTargetApplied"
  Compare To Constant1/1 -> Logical Operator/1
  Logical Operator/1 -> Switch1/2, Switch2/2
  Compare To Constant3/1 -> Logical Operator/2
  pBlowerValveOutletPlateauTarget [mmH2O]/1 -> [pBlowerValveOutletPlateauTarget]
  [pBlowerValveOutletPlateauTarget] -> Signal Conversion1/1
  Switch1/1 -> pBlowerValveOutletPlateauTargetAppliedLastCycle [mmH2O]/1, Data Store Write4/1  "pBlowerValveOutletPlateauTargetAppliedLastCycle"
  [pBlowerValveOutletPlateauTarget] -> Switch1/1

== system LIB_CycleControl/Cycle Control/Cycle Control Wrapper/Cycle pController/Pressure Target/InCycleComputation/UpdatePressureTarget ==
  NRespiratorCycleStatus [-] : Inport
  pBlowerValveOutletEndTargetApplied [mmH2O] : Inport  Port=2
  pBlowerValveOutletPlateauTargetApplied [mmH2O] : Inport  Port=3
  Enable : EnablePort
  Compare To Constant1 : simulink/Logic and Bit Operations/Compare To Constant  relop===  const=eRespiratorStates.NRespiratorInExhalation  OutDataTypeStr=boolean
  Compare To Constant2 : simulink/Logic and Bit Operations/Compare To Constant  relop===  const=eRespiratorStates.NRespiratorInInhalationPhase2  OutDataTypeStr=boolean
  Compare To Constant5 : simulink/Logic and Bit Operations/Compare To Constant  relop===  const=eRespiratorStates.NRespiratorInInhalationPhase1  OutDataTypeStr=boolean
  Constant : Constant  Value=0
  Constant1 : Constant  Value=3
  Constant2 : Constant  Value=2
  Constant3 : Constant
  Constant5 : Constant  Value=0  OutDataTypeStr=single
  Multiport Switch : MultiPortSwitch  DataPortOrder=Zero-based contiguous  Inputs=4  zeroidx=on
  Switch1 : Switch  Criteria=u2 ~= 0
      settings: AttributesFormatString=%<Criteria>
  Switch2 : Switch  Criteria=u2 ~= 0
      settings: AttributesFormatString=%<Criteria>
  Switch4 : Switch  Criteria=u2 ~= 0
      settings: AttributesFormatString=%<Criteria>
  pBlowerValveOutletTarget [mmH2O] : Outport
  wires:
  Constant3/1 -> Switch1/1
  pBlowerValveOutletPlateauTargetApplied [mmH2O]/1 -> Multiport Switch/3, Multiport Switch/2
  Compare To Constant2/1 -> Switch1/2
  Constant/1 -> Switch4/1
  pBlowerValveOutletEndTargetApplied [mmH2O]/1 -> Multiport Switch/4
  Constant2/1 -> Switch2/1
  Constant1/1 -> Switch2/3
  Switch1/1 -> Switch4/3
  Compare To Constant1/1 -> Switch2/2
  Switch2/1 -> Switch1/3
  Constant5/1 -> Multiport Switch/5
  NRespiratorCycleStatus [-]/1 -> Compare To Constant1/1, Compare To Constant2/1, Compare To Constant5/1
  Multiport Switch/1 -> pBlowerValveOutletTarget [mmH2O]/1
  Compare To Constant5/1 -> Switch4/2
  Switch4/1 -> Multiport Switch/1  "NIdxCmd"

== system LIB_CycleControl/Cycle Control/Cycle Control Wrapper/Cycle pController/Pressure processing/PPeak Computation/Peak Monitoring ==
  BInitCyclePressure [-] : Inport
  pBlowerValveOutlet [mmH2O] : Inport  Port=2
  pBlowerValveOutletPeakCurrentPrev [mmH2O] : Inport  Port=3
  Enable : EnablePort
  Constant : Constant  Value=0  OutDataTypeStr=single
  Min : MinMax  Function=max  Inputs=2
  Switch4 : Switch  Criteria=u2 ~= 0
      settings: AttributesFormatString=%<Criteria>
  pBlowerValveOutletPeakCurrent [mmH2O] : Outport
  wires:
  pBlowerValveOutletPeakCurrentPrev [mmH2O]/1 -> Min/2
  pBlowerValveOutlet [mmH2O]/1 -> Min/1
  Constant/1 -> Switch4/1
  BInitCyclePressure [-]/1 -> Switch4/2
  Min/1 -> Switch4/3
  Switch4/1 -> pBlowerValveOutletPeakCurrent [mmH2O]/1

== system LIB_CycleControl/Cycle Control/Cycle Control Wrapper/Cycle pController/Pressure processing/PPep Computation/PPep Computation ==
  BInitCyclePressure [-] : Inport
  pBlowerValveOutletLastValuesMean [mmH2O] : Inport  Port=2
  Enable : EnablePort
  Constant : Constant  Value=0  OutDataTypeStr=single
  Switch4 : Switch  Criteria=u2 ~= 0
      settings: AttributesFormatString=%<Criteria>
  pBlowerValveOutletExhalationCurrent [mmH2O] : Outport
  wires:
  pBlowerValveOutletLastValuesMean [mmH2O]/1 -> Switch4/3
  Switch4/1 -> pBlowerValveOutletExhalationCurrent [mmH2O]/1
  BInitCyclePressure [-]/1 -> Switch4/2
  Constant/1 -> Switch4/1

== system LIB_CycleControl/Cycle Control/Cycle Control Wrapper/Cycle pController/Pressure processing/PPlateau Computation/Plateau Compute ==
  BInitCyclePressure [-] : Inport
  pBlowerValveOutletLastValuesMax [mmH2O] : Inport  Port=2
  pBlowerValveOutletLastValuesMin [mmH2O] : Inport  Port=3
  pBlowerValveOutletLastValuesMean [mmH2O] : Inport  Port=4
  Enable : EnablePort
  Abs : Abs
  Constant : Constant  Value=0  OutDataTypeStr=single
  Constant2 : Constant  Value=pDiffMaxThdForPlateauPlausibility  OutDataTypeStr=single
  Relational Operator1 : RelationalOperator  Operator=<  OutDataTypeStr=boolean  RndMeth=Simplest
  Sum1 : Sum  Inputs=+-
  Switch4 : Switch  Criteria=u2 ~= 0
      settings: AttributesFormatString=%<Criteria>
  pBlowerValveOutletPlateauCurrent [mmH2O] : Outport
  BpBlowerValveOutletPlateauStabilized [-] : Outport  Port=2
  wires:
  Relational Operator1/1 -> BpBlowerValveOutletPlateauStabilized [-]/1
  Constant2/1 -> Relational Operator1/2
  Sum1/1 -> Abs/1
  Abs/1 -> Relational Operator1/1
  pBlowerValveOutletLastValuesMin [mmH2O]/1 -> Sum1/2
  pBlowerValveOutletLastValuesMax [mmH2O]/1 -> Sum1/1
  pBlowerValveOutletLastValuesMean [mmH2O]/1 -> Switch4/3
  Switch4/1 -> pBlowerValveOutletPlateauCurrent [mmH2O]/1
  BInitCyclePressure [-]/1 -> Switch4/2
  Constant/1 -> Switch4/1

== system LIB_CycleControl/Cycle Control/Cycle Control Wrapper/Cycle pController/Pressure processing/PPlateau Error Max Computation/Error Compute ==
  BInitCyclePressure [-] : Inport
  pBlowerValveOutletPlateauTargetApplied [mmH2O] : Inport  Port=2
  pBlowerValveOutlet [mmH2O] : Inport  Port=3
  pBlowerValveOutletErrorMaxCurrentPrev [mmH2O] : Inport  Port=4
  Enable : EnablePort
  Abs : Abs
  Constant : Constant  Value=0  OutDataTypeStr=single
  MinMax : MinMax  Function=max  Inputs=2
  Sum : Sum  Inputs=|+-
  Switch4 : Switch  Criteria=u2 ~= 0
      settings: AttributesFormatString=%<Criteria>
  pBlowerValveOutletErrorMaxCurrent [mmH2O] : Outport
  wires:
  MinMax/1 -> Switch4/3
  pBlowerValveOutletErrorMaxCurrentPrev [mmH2O]/1 -> MinMax/2
  Abs/1 -> MinMax/1
  Sum/1 -> Abs/1
  pBlowerValveOutlet [mmH2O]/1 -> Sum/2
  pBlowerValveOutletPlateauTargetApplied [mmH2O]/1 -> Sum/1
  Switch4/1 -> pBlowerValveOutletErrorMaxCurrent [mmH2O]/1
  BInitCyclePressure [-]/1 -> Switch4/2
  Constant/1 -> Switch4/1

== system LIB_CycleControl/Cycle Control/Cycle Control Wrapper/Cycle pController/Pressure processing/Pressure Release /Release ==
  NRespiratorCycleStatus [-] : Inport
  pBlowerValveOutletPeakCurrentPrev [mmH2O] : Inport  Port=2
  pBlowerValveOutletPlateauCurrentPrev [mmH2O] : Inport  Port=3
  pBlowerValveOutletExhalationCurrentPrev [mmH2O] : Inport  Port=4
  pBlowerValveOutletErrorMaxCurrentPrev [mmH2O] : Inport  Port=5
  BpBlowerValveOutletPlateauStabilizedPrev [-] : Inport  Port=6
  Enable : EnablePort
  Compare To Constant1 : simulink/Logic and Bit Operations/Compare To Constant  relop===  const=eRespiratorStates.NRespiratorStart  OutDataTypeStr=boolean
  Compare To Constant3 : simulink/Logic and Bit Operations/Compare To Constant  relop===  const=eRespiratorStates.NRespiratorStop  OutDataTypeStr=boolean
  Constant1 : Constant  Value=0  OutDataTypeStr=boolean
  Constant5 : Constant  Value=0  OutDataTypeStr=single
  Data Store Write1 : DataStoreWrite  DataStoreName=pBlowerValveOutletEndLastCycle
  Data Store Write2 : DataStoreWrite  DataStoreName=BpBlowerValveOutletPlateauStabilizedLastCycle
  Data Store Write3 : DataStoreWrite  DataStoreName=pBlowerValveOutletPeakLastCycle
  Data Store Write4 : DataStoreWrite  DataStoreName=pBlowerValveOutletErrorMaxLastCycle
  Data Store Write5 : DataStoreWrite  DataStoreName=pBlowerValveOutletPlateauLastCycle
  Demux : Demux
  Logical Operator : Logic  Operator=OR  AllPortsSameDT=off  OutDataTypeStr=boolean
  Mux : Mux
  Signal Conversion{1..4} (4 alike) : SignalConversion  OverrideOpt=off
  Switch1 : Switch  Criteria=u2 ~= 0
      settings: AttributesFormatString=%<Criteria>
  Switch2 : Switch  Criteria=u2 ~= 0
      settings: AttributesFormatString=%<Criteria>
  pBlowerValveOutletPeakLastCycle [mmH2O] : Outport
  pBlowerValveOutletPlateauLastCycle [mmH2O] : Outport  Port=2
  pBlowerValveOutletEndLastCycle [mmH2O] : Outport  Port=3
  pBlowerValveOutletErrorMaxLastCycle [mmH2O] : Outport  Port=4  InitialOutput=0
  wires:
  Signal Conversion4/1 -> Data Store Write4/1, pBlowerValveOutletErrorMaxLastCycle [mmH2O]/1  "pBlowerValveOutletErrorMaxLastCycle"
  Signal Conversion2/1 -> Data Store Write1/1, pBlowerValveOutletEndLastCycle [mmH2O]/1  "pBlowerValveOutletEndLastCycle"
  Signal Conversion1/1 -> pBlowerValveOutletPlateauLastCycle [mmH2O]/1, Data Store Write5/1  "pBlowerValveOutletPlateauLastCycle"
  Signal Conversion3/1 -> Data Store Write3/1, pBlowerValveOutletPeakLastCycle [mmH2O]/1  "pBlowerValveOutletPeakLastCycle"
  BpBlowerValveOutletPlateauStabilizedPrev [-]/1 -> Switch1/3
  Switch1/1 -> Data Store Write2/1  "BpBlowerValveOutletPlateauStabilizedLastCycle"
  Constant1/1 -> Switch1/1
  Demux/4 -> Signal Conversion4/1
  pBlowerValveOutletErrorMaxCurrentPrev [mmH2O]/1 -> Mux/4
  Demux/2 -> Signal Conversion1/1
  Demux/3 -> Signal Conversion2/1
  Demux/1 -> Signal Conversion3/1
  NRespiratorCycleStatus [-]/1 -> Compare To Constant3/1, Compare To Constant1/1
  Constant5/1 -> Switch2/1
  Mux/1 -> Switch2/3
  pBlowerValveOutletPeakCurrentPrev [mmH2O]/1 -> Mux/1
  pBlowerValveOutletPlateauCurrentPrev [mmH2O]/1 -> Mux/2
  pBlowerValveOutletExhalationCurrentPrev [mmH2O]/1 -> Mux/3
  Logical Operator/1 -> Switch1/2, Switch2/2
  Compare To Constant3/1 -> Logical Operator/2
  Compare To Constant1/1 -> Logical Operator/1
  Switch2/1 -> Demux/1

== system LIB_CycleControl/Cycle Control/Cycle Control Wrapper/Cycle pController/Pressure processing/Pressure recording Update/Counter ==
  Compare To Constant : simulink/Logic and Bit Operations/Compare To Constant  relop=>  const=NMaxPressureSample-1  OutDataTypeStr=boolean
  Constant : Constant  OutDataTypeStr=single
  Constant1 : Constant  Value=0  OutDataTypeStr=single
  Constant2 : Constant  Value=0  OutDataTypeStr=single
  Logical Operator : Logic  Operator=OR  AllPortsSameDT=off  OutDataTypeStr=boolean
  Sum : Sum  Inputs=|++
  Switch4 : Switch  Criteria=u2 ~= 0
      settings: AttributesFormatString=%<Criteria>
  Unit Delay : UnitDelay  SampleTime=-1
  Unit Delay1 : UnitDelay  InitialCondition=1  SampleTime=-1
  NPressureSampleIndex [-] : Outport
  wires:
  Unit Delay/1 -> Sum/2
  Constant1/1 -> Switch4/1
  Unit Delay1/1 -> Logical Operator/1
  Logical Operator/1 -> Switch4/2
  Compare To Constant/1 -> Logical Operator/2
  Constant/1 -> Sum/1
  Constant2/1 -> Unit Delay1/1
  Sum/1 -> Compare To Constant/1, Switch4/3
  Switch4/1 -> Unit Delay/1, NPressureSampleIndex [-]/1

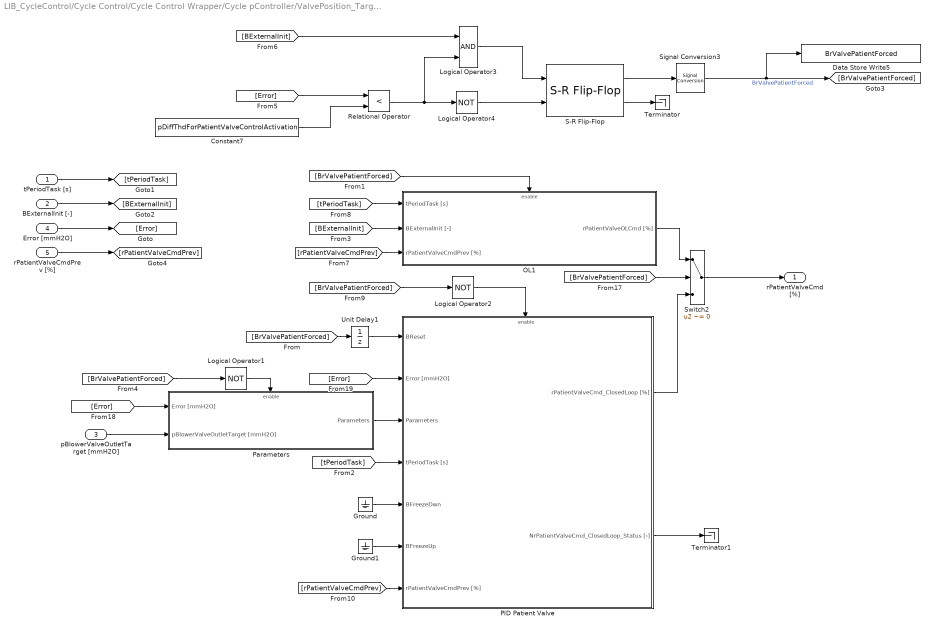
== system LIB_CycleControl/Cycle Control/Cycle Control Wrapper/Cycle pController/ValvePosition_Target/Exhalation/Patient Valve Control ==
  tPeriodTask [s] : Inport
  BExternalInit [-] : Inport  Port=2
  pBlowerValveOutletTarget [mmH2O] : Inport  Port=3
  Error [mmH2O] : Inport  Port=4
  rPatientValveCmdPrev [%] : Inport  Port=5
  Constant7 : Constant  Value=pDiffThdForPatientValveControlActivation  OutDataTypeStr=single
  Data Store Write5 : DataStoreWrite  DataStoreName=BrValvePatientForced
  Ground : Ground
  Ground1 : Ground
  Logical Operator1 : Logic  Operator=NOT  AllPortsSameDT=off  OutDataTypeStr=boolean
  Logical Operator2 : Logic  Operator=NOT  AllPortsSameDT=off  OutDataTypeStr=boolean
  Logical Operator3 : Logic  AllPortsSameDT=off  OutDataTypeStr=boolean
  Logical Operator4 : Logic  Operator=NOT  AllPortsSameDT=off  OutDataTypeStr=boolean
  OL1 : Subsystem
  PID Patient Valve : Subsystem
  Parameters : Subsystem
  Relational Operator : RelationalOperator  Operator=<  OutDataTypeStr=boolean  RndMeth=Simplest
  S-R Flip-Flop : simulink_extras/Flip Flops/S-R Flip-Flop  initial_condition=0
  Signal Conversion3 : SignalConversion  OverrideOpt=off
  Switch2 : Switch  Criteria=u2 ~= 0
      settings: AttributesFormatString=%<Criteria>
  Terminator : Terminator
  Terminator1 : Terminator
  Unit Delay1 : UnitDelay  SampleTime=-1
  rPatientValveCmd [%] : Outport
  wires:
  Signal Conversion3/1 -> [BrValvePatientForced], Data Store Write5/1  "BrValvePatientForced"
  pBlowerValveOutletTarget [mmH2O]/1 -> Parameters/2(pBlowerValveOutletTarget [mmH2O])
  Constant7/1 -> Relational Operator/2
  [rPatientValveCmdPrev] -> PID Patient Valve/7(rPatientValveCmdPrev [%])
  [BrValvePatientForced] -> Logical Operator2/1
  Switch2/1 -> rPatientValveCmd [%]/1
  [rPatientValveCmdPrev] -> OL1/3(rPatientValveCmdPrev [%])
  [BExternalInit] -> OL1/2(BExternalInit [-])
  [tPeriodTask] -> OL1/1(tPeriodTask [s])
  OL1/1(rPatientValveOLCmd [%]) -> Switch2/1
  [BrValvePatientForced] -> OL1/Enable
  Ground1/1 -> PID Patient Valve/6(BFreezeUp)
  Ground/1 -> PID Patient Valve/5(BFreezeDwn)
  Unit Delay1/1 -> PID Patient Valve/1(BReset)
  rPatientValveCmdPrev [%]/1 -> [rPatientValveCmdPrev]
  [tPeriodTask] -> PID Patient Valve/4(tPeriodTask [s])
  [Error] -> PID Patient Valve/2(Error [mmH2O])
  [Error] -> Parameters/1(Error [mmH2O])
  PID Patient Valve/1(rPatientValveCmd_ClosedLoop [%]) -> Switch2/3
  PID Patient Valve/2(NrPatientValveCmd_ClosedLoop_Status [-]) -> Terminator1/1
  Parameters/1(Parameters) -> PID Patient Valve/3(Parameters)
  Logical Operator4/1 -> S-R Flip-Flop/2
  Relational Operator/1 -> Logical Operator3/2, Logical Operator4/1
  S-R Flip-Flop/1 -> Signal Conversion3/1
  S-R Flip-Flop/2 -> Terminator/1
  Logical Operator3/1 -> S-R Flip-Flop/1
  [BrValvePatientForced] -> Switch2/2
  [Error] -> Relational Operator/1
  BExternalInit [-]/1 -> [BExternalInit]
  tPeriodTask [s]/1 -> [tPeriodTask]
  Error [mmH2O]/1 -> [Error]
  Logical Operator2/1 -> PID Patient Valve/Enable
  [BrValvePatientForced] -> Unit Delay1/1
  [BExternalInit] -> Logical Operator3/1
  [BrValvePatientForced] -> Logical Operator1/1
  Logical Operator1/1 -> Parameters/Enable

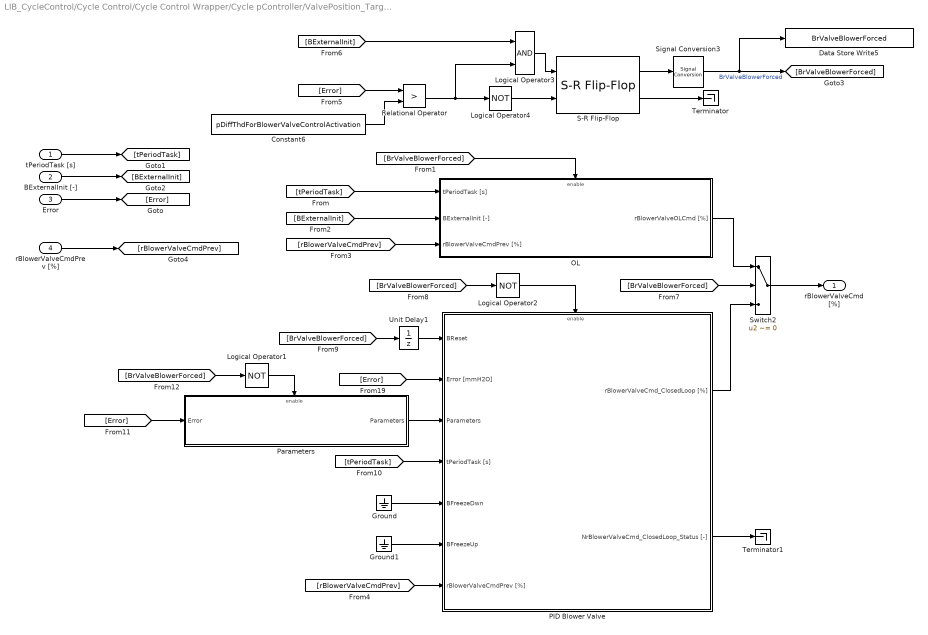
== system LIB_CycleControl/Cycle Control/Cycle Control Wrapper/Cycle pController/ValvePosition_Target/Inhalation/Blower Valve Control ==
  tPeriodTask [s] : Inport
  BExternalInit [-] : Inport  Port=2
  Error : Inport  Port=3
  rBlowerValveCmdPrev [%] : Inport  Port=4
  Constant6 : Constant  Value=pDiffThdForBlowerValveControlActivation  OutDataTypeStr=single
  Data Store Write5 : DataStoreWrite  DataStoreName=BrValveBlowerForced
  Ground : Ground
  Ground1 : Ground
  Logical Operator1 : Logic  Operator=NOT  AllPortsSameDT=off  OutDataTypeStr=boolean
  Logical Operator2 : Logic  Operator=NOT  AllPortsSameDT=off  OutDataTypeStr=boolean
  Logical Operator3 : Logic  AllPortsSameDT=off  OutDataTypeStr=boolean
  Logical Operator4 : Logic  Operator=NOT  AllPortsSameDT=off  OutDataTypeStr=boolean
  OL : Subsystem
  PID Blower Valve : Subsystem
  Parameters : Subsystem
  Relational Operator : RelationalOperator  Operator=>  OutDataTypeStr=boolean  RndMeth=Simplest
  S-R Flip-Flop : simulink_extras/Flip Flops/S-R Flip-Flop  initial_condition=0
  Signal Conversion3 : SignalConversion  OverrideOpt=off
  Switch2 : Switch  Criteria=u2 ~= 0
      settings: AttributesFormatString=%<Criteria>
  Terminator : Terminator
  Terminator1 : Terminator
  Unit Delay1 : UnitDelay  SampleTime=-1
  rBlowerValveCmd [%] : Outport
  wires:
  Signal Conversion3/1 -> [BrValveBlowerForced], Data Store Write5/1  "BrValveBlowerForced"
  Constant6/1 -> Relational Operator/2
  [BrValveBlowerForced] -> Logical Operator2/1
  [rBlowerValveCmdPrev] -> PID Blower Valve/7(rBlowerValveCmdPrev [%])
  Switch2/1 -> rBlowerValveCmd [%]/1
  [rBlowerValveCmdPrev] -> OL/3(rBlowerValveCmdPrev [%])
  [BExternalInit] -> OL/2(BExternalInit [-])
  [tPeriodTask] -> OL/1(tPeriodTask [s])
  [BrValveBlowerForced] -> Switch2/2
  OL/1(rBlowerValveOLCmd [%]) -> Switch2/1
  [BrValveBlowerForced] -> OL/Enable
  Ground1/1 -> PID Blower Valve/6(BFreezeUp)
  Ground/1 -> PID Blower Valve/5(BFreezeDwn)
  Unit Delay1/1 -> PID Blower Valve/1(BReset)
  rBlowerValveCmdPrev [%]/1 -> [rBlowerValveCmdPrev]
  [tPeriodTask] -> PID Blower Valve/4(tPeriodTask [s])
  [Error] -> PID Blower Valve/2(Error [mmH2O])
  PID Blower Valve/1(rBlowerValveCmd_ClosedLoop [%]) -> Switch2/3
  PID Blower Valve/2(NrBlowerValveCmd_ClosedLoop_Status [-]) -> Terminator1/1
  Parameters/1(Parameters) -> PID Blower Valve/3(Parameters)
  Logical Operator4/1 -> S-R Flip-Flop/2
  Relational Operator/1 -> Logical Operator4/1, Logical Operator3/2
  S-R Flip-Flop/1 -> Signal Conversion3/1
  S-R Flip-Flop/2 -> Terminator/1
  Logical Operator3/1 -> S-R Flip-Flop/1
  [BExternalInit] -> Logical Operator3/1
  [Error] -> Relational Operator/1
  BExternalInit [-]/1 -> [BExternalInit]
  tPeriodTask [s]/1 -> [tPeriodTask]
  Error/1 -> [Error]
  [BrValveBlowerForced] -> Unit Delay1/1
  Logical Operator2/1 -> PID Blower Valve/Enable
  [Error] -> Parameters/1(Error)
  [BrValveBlowerForced] -> Logical Operator1/1
  Logical Operator1/1 -> Parameters/Enable

== system LIB_CycleControl/Cycle Control/Cycle Control Wrapper/Cycle pController/ValvePosition_Target/Exhalation/Patient Valve Control/OL1 ==
  tPeriodTask [s] : Inport
  BExternalInit [-] : Inport  Port=2
  rPatientValveCmdPrev [%] : Inport  Port=3
  Enable : EnablePort
  Constant2 : Constant  Value=100  OutDataTypeStr=single
  Constant5 : Constant  Value=tPatientValveOpen  OutDataTypeStr=single
  Gain : Gain  Gain=-1
  Product : Product  Inputs=*/
  Product1 : Product  Inputs=*/
  Rate Lmiter : Subsystem  mask(Rate Limiter Dynamic){}
      mask help: Simulink:masks:RateLimiterDynamic_MD
  Switch3 : Switch  Criteria=u2 ~= 0
      settings: AttributesFormatString=%<Criteria>
  Unit Delay1 : UnitDelay  SampleTime=-1
  rPatientValveOLCmd [%] : Outport
  wires:
  Constant5/1 -> Product1/2, Product/2
  Unit Delay1/1 -> Switch3/3
  tPeriodTask [s]/1 -> Rate Lmiter/1(tPeriodTask [s])
  BExternalInit [-]/1 -> Switch3/2
  Product1/1 -> Rate Lmiter/4(lo)
  Product/1 -> Rate Lmiter/2(up)
  rPatientValveCmdPrev [%]/1 -> Switch3/1
  Switch3/1 -> Rate Lmiter/5(Y(k-1))
  Rate Lmiter/1(Y(k)) -> Unit Delay1/1, rPatientValveOLCmd [%]/1
  Constant2/1 -> Gain/1, Product/1, Rate Lmiter/3(u)
  Gain/1 -> Product1/1
